simulink model "SIMULINK_DUE_UART_TALK_1Hz_48bytes"  (R2022a)
settings: Solver=ode3  StartTime=0.0  StopTime=60  RelTol=1e-3  EnableMultiTasking=on
libraries: arduinolib x5, svdutilitieslib x2
settings Model: FPTRunName=Active  ExtModeTrigDuration=2  Creator=Rafael  LastModifiedBy=Rafael
settings SolverCC: AlgebraicLoopSolver=TrustRegion  AutoInsertRateTranBlk=on
settings DataIOCC: LimitDataPoints=on  SaveFormat=Array
settings OptimizationCC: DefaultParameterBehavior=Inlined  ExpressionDepthLimit=2147483647  LifeSpan=Inf  MaxStackSize=64
settings DebuggingCC: UnderspecifiedInitializationDetection=Classic  MergeDetectMultiDrivingBlocksExec=none  FcnCallInpInsideContextMsg=warning  UnconnectedInputMsg=warning  UnconnectedOutputMsg=warning  UnconnectedLineMsg=warning  AllowSymbolicDim=off  StateNameClashWarn=warning  SFUnexpectedBacktrackingDiag=warning  SFNoUnconditionalDefaultTransitionDiag=warning  SFExecutionAtInitializationDiag=none  SFMachineParentedDataDiag=warning  ArithmeticOperatorsInVariantConditions=warning
settings HardwareCC: ProdBitPerPointer=32  ProdBitPerSizeT=32  ProdBitPerPtrDiffT=32  ProdLargestAtomicInteger=Long  ProdLargestAtomicFloat=Double  ProdWordSize=32  ProdHWDeviceType=ARM Compatible->ARM Cortex
settings ModelReferenceCC: PropagateSignalLabelsOutOfModel=off
settings SFSimCC: SimUseLocalCustomCode=off  CustomCodeUndefinedFunction=UseInterfaceOnly
settings RTWCC: SystemTargetFile=ert.tlc  HardwareBoard=Arduino Due  TemplateMakefile=ert_default_tmf  GenerateReport=on  RTWVerbose=off  RTWUseLocalCustomCode=off  Toolchain=Arduino ARM  BuildConfiguration=Faster Runs  LaunchReport=on
settings CodeAppCC: ForceParamTrailComments=on  OperatorAnnotations=on  StateflowObjectComments=on  MATLABSourceComments=on
settings ERTTargetCC: MultiwordLength=2048  ERTCustomFileBanners=off  SupportContinuousTime=on  SupportNonInlinedSFcns=on  RemoveResetFunc=off  SupportVariableSizeSignals=on  ModelStepFunctionPrototypeControlCompliant=off  ExtModeTransport=3  ExtModeStaticAlloc=on  ExtModeStaticAllocSize=24576  ExtModeMexFile=ext_xcp  ExtModeIntrfLevel=Level2 - Open
settings ConfigComp: CovMetricSettings=dw  CovSaveCumulativeToWorkspaceVar=on  CovSaveSingleToWorkspaceVar=on  CovExternalEMLEnable=off  CovSFcnEnable=off

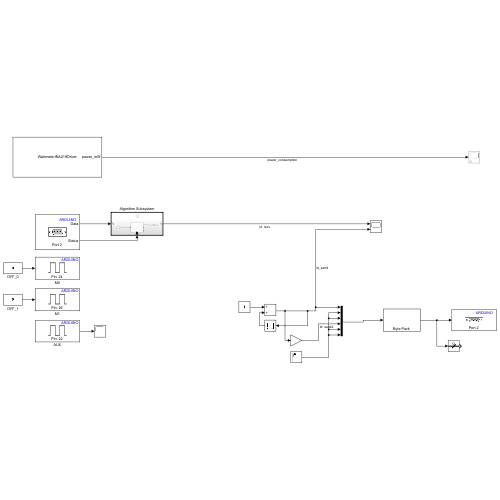
[thumbnail: Simulink's stored preview of the top-level diagram]
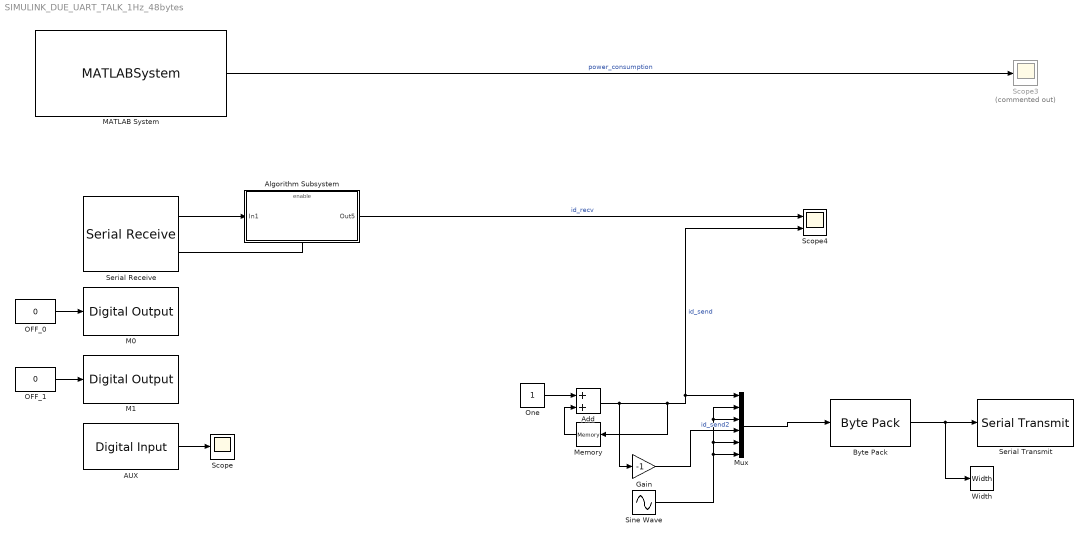
== system SIMULINK_DUE_UART_TALK_1Hz_48bytes ==
  AUX : arduinolib/Digital Input  pinNumber=22  mode=Default  Direction=input  SampleTime=0.01  blockPlatform=arduino
  Add : Sum
  Algorithm Subsystem : Subsystem
  Byte Pack : svdutilitieslib/Byte Pack  maskPackedDataType=uint8  datatypes={'double'}  byteAlign=8  blockPlatform=arduinoert
      settings: SourceProductBaseCode=ANDROID,ARDUINO,ML_ARDUINO,ECCORTEXA,ECCORTEXR,SC_BEAGLEBONE_BLUE,EC_FREEDOM_BOARD,EC_FRDM_K64F,INTEL_BLOCKSET,MICROBIT,NUCLEO,NVIDIA,PX4AUTOPILOTS,RASPPIIO,STMICRODIS,TIC2000,XILINX_BLOCKSET
  Gain : Gain  Gain=-1
  M0 : arduinolib/Digital Output  pinNumber=24  Direction=output  blockPlatform=arduino
  M1 : arduinolib/Digital Output  pinNumber=26  Direction=output  blockPlatform=arduino
  MATLAB System : MATLABSystem  System=WattmeterINA219Driver  id=0  address=40  SampleTime=0.01
      mask Type: WattmeterINA219Driver
      mask Display:
      | disp('WattmeterINA219Driver');
      | port_label('output',1,'power_mW');
  Memory : Memory  InheritSampleTime=on
  Mux : Mux  Inputs=6
  OFF_0 : Constant  Value=0  SampleTime=-1
  OFF_1 : Constant  Value=0  SampleTime=-1
  One : Constant  OutDataTypeStr=Inherit: Inherit via back propagation  SampleTime=1
  Scope : Scope
  Scope3 : Scope  Commented=on
  Scope4 : Scope  NumInputPorts=2
  Serial Receive : arduinolib/Serial Receive  isARMArch=on  portNumber=2  DataType=uint8  Datalength=24  SampleTime=0.001  showOutStatus=on  blockPlatform=arduino
      settings: SourceProductBaseCode=ARDUINO
  Serial Transmit : arduinolib/Serial Transmit  portNumber=2  sendmode=write  sendformat=Decimal  floatprecision=2  blockPlatform=arduino
  Sine Wave : Sin  Frequency=0.2  SampleTime=1
  Width : Width
  wires:
  OFF_0/1 -> M0/1
  OFF_1/1 -> M1/1
  Serial Receive/1 -> Algorithm Subsystem/1(In1)
  AUX/1 -> Scope/1
  Serial Receive/2 -> Algorithm Subsystem/Enable
  MATLAB System/1 -> Scope3/1  "power_consumption"
  One/1 -> Add/1
  Add/1 -> Gain/1, Memory/1, Scope4/2, Mux/1  "id_send"
  Memory/1 -> Add/2
  Algorithm Subsystem/1(Out5) -> Scope4/1  "id_recv"
  Byte Pack/1 -> Serial Transmit/1, Width/1
  Mux/1 -> Byte Pack/1
  Gain/1 -> Mux/4  "id_send2"
  Sine Wave/1 -> Mux/2, Mux/3, Mux/5, Mux/6

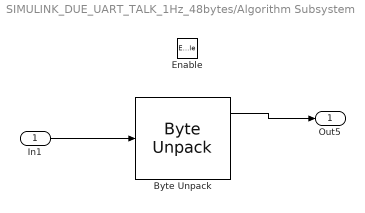
== system SIMULINK_DUE_UART_TALK_1Hz_48bytes/Algorithm Subsystem ==
  In1 : Inport
  Enable : EnablePort
  Byte Unpack : svdutilitieslib/Byte Unpack  dimensions={1,1,1}  datatypes={'double','double','double'}  byteAlign=8  blockPlatform=arduinoert
      settings: SourceProductBaseCode=ANDROID,ARDUINO,ML_ARDUINO,ECCORTEXA,ECCORTEXR,SC_BEAGLEBONE_BLUE,EC_FREEDOM_BOARD,EC_FRDM_K64F,INTEL_BLOCKSET,MICROBIT,NUCLEO,NVIDIA,PX4AUTOPILOTS,RASPPIIO,STMICRODIS,TIC2000,XILINX_BLOCKSET
  Out5 : Outport  VectorParamsAs1DForOutWhenUnconnected=off
  wires:
  In1/1 -> Byte Unpack/1
  Byte Unpack/1 -> Out5/1
